simulink model "merge_variable_grain"  (R2023b)
settings: Solver=FixedStepAuto  StartTime=0.0  StopTime=inf  RelTol=1e-3
InitFcn:
  | myapp = app3;
StartFcn:
  | blk = 'merge_variable_grain/Biquad Filtering/speed_disp';
  | event = 'PostOutputs';
  | listener = @(app,event) updateGUI(myapp);
  | h = add_exec_event_listener(blk, event, listener);
StopFcn:
  | delete(myapp)
values from neighbouring files (symbols this model uses):
  audio_1 = audio_2_nr    [inizio.m]    (also in load_preset_audio.m; resample_workspace.m = resample(audio_1, f_resample, fs))
  audio_2 = audio_2_nr    [inizio.m]    (also in load_preset_audio.m; resample_workspace.m = resample(audio_2, f_resample, fs2))
  audio_3 = audio_3_nr    [inizio.m]    (also in load_preset_audio.m; resample_workspace.m = resample(audio_3, f_resample, fs3))
  fs = f_resample    [inizio.m]    (also in load_preset_audio.m; resample_workspace.m)
undefined symbols (not defined in the file or in its folder): canChannel, DiscIntNeverNeededParam
libraries: canmsglib x14, canlib x9, dspfdesign x9, dspsnks4 x1, audiofilters x1, audiodynamicrange x1, simulink x1
settings Model: Creator=The MathWorks, Inc.  LastModifiedBy=giorg
settings SolverCC: AlgebraicLoopSolver=TrustRegion
settings DataIOCC: SaveFormat=Array  ReturnWorkspaceOutputs=off
settings DebuggingCC: UnconnectedInputMsg=warning  UnconnectedOutputMsg=warning  UnconnectedLineMsg=warning  ArithmeticOperatorsInVariantConditions=warning
settings ModelReferenceCC: EnableRefExpFcnMdlSchedulingChecks=on
settings SFSimCC: SimUseLocalCustomCode=off  CustomCodeUndefinedFunction=UseInterfaceOnly
settings RTWCC: RTWUseLocalCustomCode=off

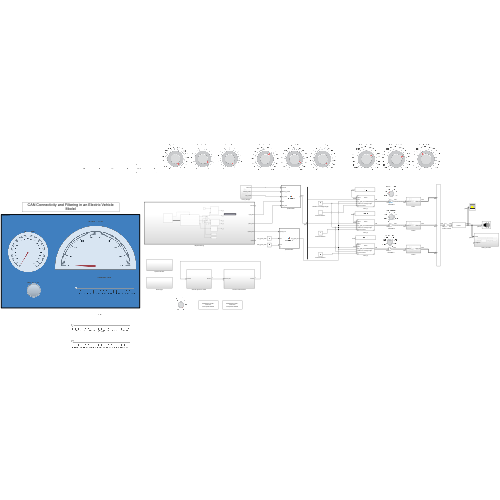
[thumbnail: Simulink's stored preview of the top-level diagram]
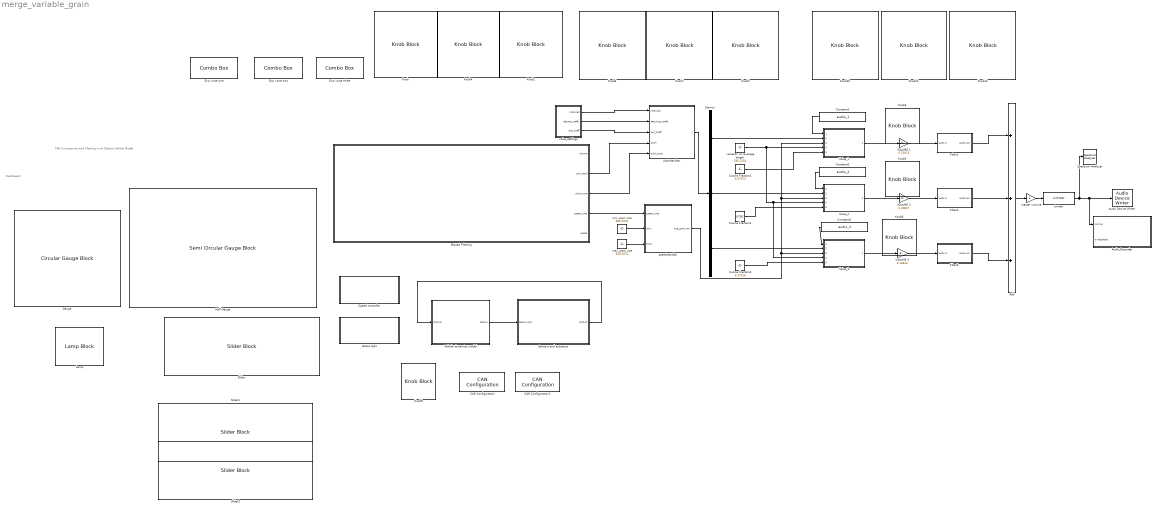
== system merge_variable_grain ==
  note: Dashboard
  note: CAN Connectivity and Filtering in an Electric Vehicle Model
  Add : Sum  Inputs=+++
  Audio Device Writer : dspsnks4/Audio Device Writer  Driver=DirectSound  Device=Default  InheritSampleRate=off  SampleRate=fs  BitDepth=16-bit integer  BufferSize=4096  NumBuffers=10  DefaultOutputChannelMapping=on  OutputChannelMapping=1:2  OutputNumUnderrunSamples=off  DriverIdx=1  DeviceWarnFlag=''
  Audio_Recorder : Subsystem
  Biquad Filtering : Subsystem  TreatAsAtomicUnit=on
  Brake light : Subsystem
  CAN Configuration : canlib/CAN Configuration  BlockHandle=142.0001  Device=MathWorks Virtual 1 (Channel 1)  DeviceMenu=MathWorks Virtual 1 (Channel 1)  ObjConstructor=canChannel('MathWorks', 'Virtual 1', 1)  BusSpeed=500000  EnableBitParameters=off  AckMode=Normal
  CAN Configuration1 : canlib/CAN Configuration  BlockHandle=143.0001  Device=MathWorks Virtual 1 (Channel 2)  DeviceMenu=MathWorks Virtual 1 (Channel 2)  ObjConstructor=canChannel('MathWorks', 'Virtual 1', 2)  BusSpeed=500000  EnableBitParameters=off  AckMode=Normal
  Constant1 : Constant  Value=audio_1
  Constant2 : Constant  Value=audio_2
  Constant3 : Constant  Value=audio_3
  Cosine Fraction1 : Constant  Value=0.67973
  Cosine Fraction2 : Constant  Value=0.7202
  Cosine Fraction3 : Constant  Value=0.37916
  Demux : Demux  Outputs=3
  Exp voice one : ComboBox  LabelPosition=Hide  SelectedLabel=Linear
      settings: Values={{'Linear', 'Quadratic', 'Cubic'}, [1 2 3]}
  Exp voice three : ComboBox  LabelPosition=Hide  SelectedLabel=Linear
      settings: Values={{'Linear', 'Quadratic', 'Cubic'}, [1 2 3]}
  Exp voice two : ComboBox  LabelPosition=Hide  SelectedLabel=Linear
      settings: Values={{'Linear', 'Quadratic', 'Cubic'}, [1 2 3]}
  Filter1 : Subsystem
  Filter2 : Subsystem
  Filter3 : Subsystem
  Gauge : CircularGaugeBlock  ScaleMax=200  TickInterval=10
  Half Gauge : SemiCircularGaugeBlock  ScaleMax=9000  TickInterval=1000
  Knob{,3,5,8,10..12} (7 alike) : KnobBlock  ScaleMax=1
  Knob1 : KnobBlock  ScaleMax=12  TickInterval=1
  Knob2 : KnobBlock  ScaleMin=30  ScaleMax=200
  Knob4 : KnobBlock  ScaleMin=-12  ScaleMax=2  TickInterval=1
  Knob6 : KnobBlock  ScaleMin=100  ScaleMax=1000
  Knob7 : KnobBlock  ScaleMin=300  ScaleMax=1000
  Knob9 : KnobBlock  ScaleMin=0.5  ScaleMax=1
  Lamp : LampBlock
  Limiter : audiodynamicrange/Limiter  ThresholdPort=off  Threshold=0  KneeWidthPort=off  KneeWidth=0.0  AttackTimePort=off  AttackTime=0.0  ReleaseTimePort=off  ReleaseTime=0.120  MakeUpGainMode=Property  MakeUpGain=0.0  InheritSampleRate=off  SampleRate=fs  outputGain=off  EnableSidechain=off  SimulateUsing=Code generation
  Sensors and actuators : Subsystem
  Slider : SliderBlock  ScaleMax=200
  Slider1 : SliderBlock  ScaleMax=1
  Slider2 : SliderBlock  ScaleMax=1
  Spectrum Analyzer : SpectrumAnalyzer  WindowPosition=[309.000000,143.000000,800.000000,500.000000,]  Visible=on  ScopeFrameLocation=window  SampleRateSource=Property  SampleRate=44.1e3  PlotAsTwoSidedSpectrum=off  FrequencyScale=Log  FrequencySpan=Start and stop frequencies  StartFrequency=20  StopFrequency=20e3  SpectrumUnits=dBW  YLimits=[-213.94607708,3.88433958]  SelectedToolstripTab=spectrumAnalyzerToolstrip.spectrumTab
  Speed controller : Subsystem
  VOLUME 1 : Gain  Gain=0.31015
  VOLUME 2 : Gain  Gain=0.30827
  VOLUME 3 : Gain  Gain=0.13644
  Vehicle dynamics model : Subsystem
  Voice_1 : Subsystem  ReferencedSubsystem=Voice  rng_seeds=rng_seeds_thread_1  sample_dim_f=max_s1
  Voice_2 : Subsystem  ReferencedSubsystem=Voice  rng_seeds=rng_seeds_thread_2  sample_dim_f=max_s2
  Voice_3 : Subsystem  ReferencedSubsystem=Voice  rng_seeds=rng_seeds_thread_3  sample_dim_f=max_s3
  master volume : Gain
  max_grain_size : Constant  Value=928.4031
  min_grain_size : Constant  Value=665.0231
  pitchHandler : MATLAB Function  TreatAsAtomicUnit=on
  speedHandler : MATLAB Function  TreatAsAtomicUnit=on  mask{fs=fs}
      mask prompts: fs "sampling frequency"
  variation on average length : Constant  Value=195.2254
  voice_settings : Subsystem
  wires:
  Vehicle dynamics model/1(Sensor) -> Sensors and actuators/1(Sensor port)
  Sensors and actuators/1(Control) -> Vehicle dynamics model/1(Control)
  pitchHandler/1(y) -> Demux/1
  Add/1 -> master volume/1
  Voice_1/1 -> VOLUME 1/1
  Demux/1 -> Voice_1/2
  Voice_3/1 -> VOLUME 3/1
  Constant1/1 -> Voice_1/1
  speedHandler/1(avg_grain_len) -> Voice_2/3, Voice_1/3, Voice_3/3
  Biquad Filtering/2(rpm_pitch) -> pitchHandler/4(pitch)
  VOLUME 1/1 -> Filter1/1(audio in)
  VOLUME 3/1 -> Filter3/1(audio in)
  VOLUME 2/1 -> Filter2/1(audio in)
  Demux/2 -> Voice_2/2
  Demux/3 -> Voice_3/2
  Biquad Filtering/3(pitch_tune) -> pitchHandler/5(pitch_tune)
  voice_settings/1(intervals) -> pitchHandler/1(intervals)
  voice_settings/2(detune_coeffs) -> pitchHandler/2(detuning_coeffs)
  Filter1/1(audio out) -> Add/1
  Filter2/1(audio out) -> Add/2
  Filter3/1(audio out) -> Add/3
  min_grain_size/1 -> speedHandler/2(tmin)
  Biquad Filtering/4(speed_tune) -> speedHandler/1(speed_tune)
  max_grain_size/1 -> speedHandler/3(tmax)
  variation on average length/1 -> Voice_3/4, Voice_2/4, Voice_1/4
  Constant3/1 -> Voice_3/1
  voice_settings/3(exp_coeff) -> pitchHandler/3(exp_coeff)
  Voice_2/1 -> VOLUME 2/1
  Constant2/1 -> Voice_2/1
  Cosine Fraction1/1 -> Voice_1/5
  Cosine Fraction2/1 -> Voice_2/5
  Cosine Fraction3/1 -> Voice_3/5
  master volume/1 -> Limiter/1
  Limiter/1 -> Spectrum Analyzer/1, Audio_Recorder/1(normal), Audio Device Writer/1

== system merge_variable_grain/Audio_Recorder ==
  normal : Inport
  a-weighted : Inport  Port=2
  Reshape : Reshape
  Reshape1 : Reshape
  To Workspace : ToWorkspace  VariableName=audio_output  SaveFormat=Structure  SampleTime=-1
      settings: Save2DSignal=2-D array (concatenate along first dimension)
  To Workspace1 : ToWorkspace  VariableName=audio_output_A  SaveFormat=Structure  SampleTime=-1
      settings: Save2DSignal=2-D array (concatenate along first dimension)
  Weighting Filter : audiofilters/Weighting Filter  Method=A-weighting  InheritSampleRate=off  SampleRate=fs  SimulateUsing=Code generation  WorkspaceVariableName=myFilt  OverwriteExportVariable=on  MaskClassType=No mask
  wires:
  Weighting Filter/1 -> Reshape/1
  normal/1 -> Reshape1/1
  Reshape1/1 -> To Workspace/1
  a-weighted/1 -> Weighting Filter/1
  Reshape/1 -> To Workspace1/1

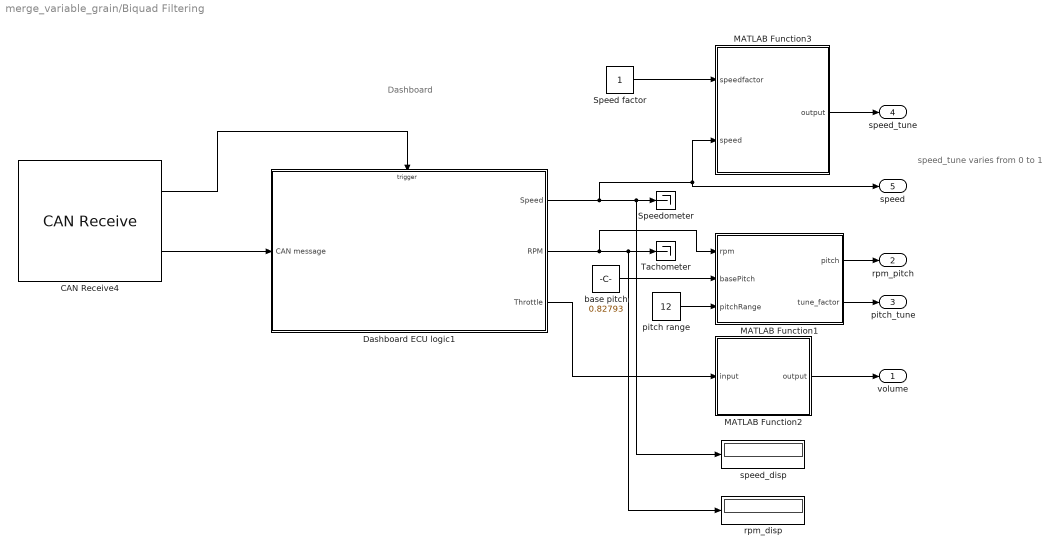
== system merge_variable_grain/Biquad Filtering ==
  note: speed_tune varies from 0 to 1
  note: Dashboard
  CAN Receive4 : canlib/CAN Receive  BlockHandle=19.0001  Device=MathWorks Virtual 1 (Channel 1)  DeviceMenu=MathWorks Virtual 1 (Channel 1)  ObjConstructor=canChannel('MathWorks', 'Virtual 1', 1)  EnableStandardIDsFilter=off  StdIDsCombo=Block all  StandardIDs=0  EnableExtendedIDsFilter=off  ExtIDsCombo=Allow all  ExtendedIDs=[50 100]  SampleTime=0.01  MsgsPerTimestep=all  InternalFilterUpdateStatus=on  BusOutput=on
  Dashboard ECU logic1 : Subsystem  TreatAsAtomicUnit=on
  MATLAB Function1 : MATLAB Function  TreatAsAtomicUnit=on
  MATLAB Function2 : MATLAB Function  TreatAsAtomicUnit=on
  MATLAB Function3 : MATLAB Function  TreatAsAtomicUnit=on
  Speed factor : Constant
  Speedometer : Terminator
  Tachometer : Terminator
  base pitch : Constant  Value=0.82793
  pitch range : Constant  Value=12
  rpm_disp : Display
  speed_disp : Display
  volume : Outport
  rpm_pitch : Outport  Port=2
  pitch_tune : Outport  Port=3
  speed_tune : Outport  Port=4
  speed : Outport  Port=5
  wires:
  Dashboard ECU logic1/3(Throttle) -> MATLAB Function2/1(input)
  MATLAB Function2/1(output) -> volume/1
  Dashboard ECU logic1/1(Speed) -> MATLAB Function3/2(speed), speed/1, speed_disp/1, Speedometer/1
  CAN Receive4/2 -> Dashboard ECU logic1/1(CAN message)
  Dashboard ECU logic1/2(RPM) -> rpm_disp/1, Tachometer/1, MATLAB Function1/1(rpm)
  CAN Receive4/1 -> Dashboard ECU logic1/Trigger
  MATLAB Function1/1(pitch) -> rpm_pitch/1
  MATLAB Function3/1(output) -> speed_tune/1
  Speed factor/1 -> MATLAB Function3/1(speedfactor)
  base pitch/1 -> MATLAB Function1/2(basePitch)
  MATLAB Function1/2(tune_factor) -> pitch_tune/1
  pitch range/1 -> MATLAB Function1/3(pitchRange)

== system merge_variable_grain/Brake light ==
  note: Brake light
  Brake light : Terminator
  Brake light ECU logic : Subsystem  TreatAsAtomicUnit=on
  CAN Receive : canlib/CAN Receive  BlockHandle=137.0001  Device=MathWorks Virtual 1 (Channel 2)  DeviceMenu=MathWorks Virtual 1 (Channel 2)  ObjConstructor=canChannel('MathWorks', 'Virtual 1', 2)  EnableStandardIDsFilter=off  StdIDsCombo=Allow all  StandardIDs=0  EnableExtendedIDsFilter=off  ExtIDsCombo=Allow all  ExtendedIDs=0  SampleTime=0.01  MsgsPerTimestep=all  InternalFilterUpdateStatus=on  BusOutput=on
  wires:
  CAN Receive/1 -> Brake light ECU logic/Trigger
  CAN Receive/2 -> Brake light ECU logic/1(CAN message)
  Brake light ECU logic/1(Brake status) -> Brake light/1

== system merge_variable_grain/Filter1 ==
  audio in : Inport
  Subsystem : Subsystem
  bandwidth : Constant  Value=999
  center_freq : Constant  Value=500
  cutoff_freq : Constant  Value=10000
  switch : Constant
  audio out : Outport
  wires:
  center_freq/1 -> Subsystem/1(In1)
  bandwidth/1 -> Subsystem/2(In2)
  audio in/1 -> Subsystem/3(In3)
  cutoff_freq/1 -> Subsystem/4(In4)
  switch/1 -> Subsystem/5(c)
  Subsystem/1(y) -> audio out/1

== system merge_variable_grain/Filter2 ==
  audio in : Inport
  Subsystem : Subsystem
  bandwidth : Constant  Value=950
  center_freq : Constant  Value=1000
  cutoff_freq : Constant  Value=10000
  switch : Constant
  audio out : Outport
  wires:
  Subsystem/1(y) -> audio out/1
  switch/1 -> Subsystem/5(c)
  cutoff_freq/1 -> Subsystem/4(In4)
  audio in/1 -> Subsystem/3(In3)
  bandwidth/1 -> Subsystem/2(In2)
  center_freq/1 -> Subsystem/1(In1)

== system merge_variable_grain/Filter3 ==
  audio in : Inport
  Subsystem : Subsystem
  bandwidth : Constant  Value=500
  center_freq : Constant  Value=500
  cutoff_freq : Constant  Value=10000
  switch : Constant
  audio out : Outport
  wires:
  center_freq/1 -> Subsystem/1(In1)
  bandwidth/1 -> Subsystem/2(In2)
  audio in/1 -> Subsystem/3(In3)
  cutoff_freq/1 -> Subsystem/4(In4)
  switch/1 -> Subsystem/5(c)
  Subsystem/1(y) -> audio out/1

== system merge_variable_grain/Sensors and actuators ==
  note: Sensors and actuators
  Sensor port : Inport
  Actuators : Subsystem
  CAN Receive interface : Subsystem
  CAN Transmit interface : Subsystem
  Sensors : Subsystem
  Control : Outport  VectorParamsAs1DForOutWhenUnconnected=off
  wires:
  Sensor port/1 -> Sensors/1(Sensor port)
  Sensors/1(RPM) -> CAN Transmit interface/2(RPM)
  Sensors/2(Speed) -> CAN Transmit interface/3(Speed)
  Actuators/1(Control) -> Control/1
  Actuators/2(Brake status) -> CAN Transmit interface/1(Brake status)
  CAN Receive interface/1(Throttle command) -> Actuators/1(Throttle command)
  CAN Receive interface/2(Brake command) -> Actuators/2(Brake command)

== system merge_variable_grain/Speed controller ==
  note: Speed controller
  CAN Receive : canlib/CAN Receive  BlockHandle=455.0001  Device=MathWorks Virtual 1 (Channel 2)  DeviceMenu=MathWorks Virtual 1 (Channel 2)  ObjConstructor=canChannel('MathWorks', 'Virtual 1', 2)  EnableStandardIDsFilter=off  StdIDsCombo=Allow all  StandardIDs=0  EnableExtendedIDsFilter=off  ExtIDsCombo=Allow all  ExtendedIDs=0  SampleTime=0.01  MsgsPerTimestep=all  InternalFilterUpdateStatus=on  BusOutput=on
  Speed controller ECU logic : Subsystem  TreatAsAtomicUnit=on
  wires:
  CAN Receive/1 -> Speed controller ECU logic/Trigger
  CAN Receive/2 -> Speed controller ECU logic/1(CAN message)

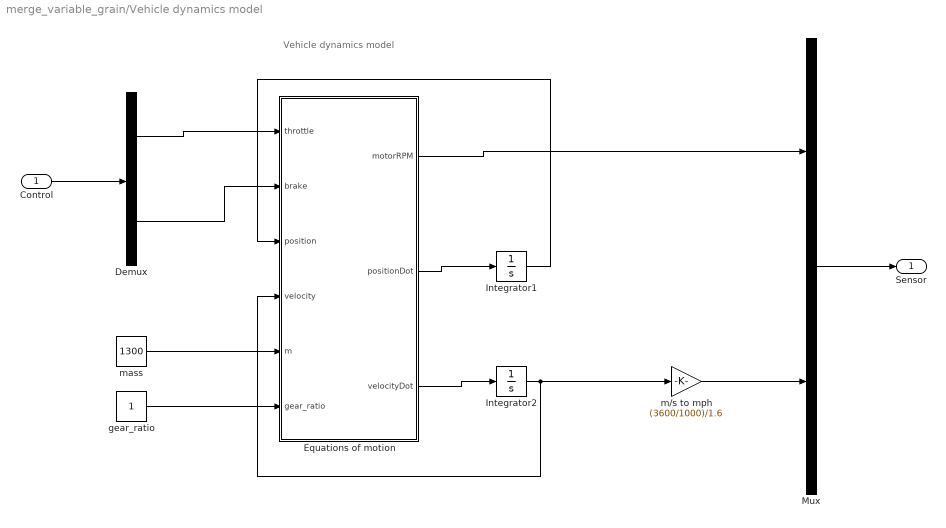
== system merge_variable_grain/Vehicle dynamics model ==
  note: Vehicle dynamics model
  Control : Inport
  Demux : Demux  Outputs=2
  Equations of motion : MATLAB Function  TreatAsAtomicUnit=on
  Integrator1 : Integrator
  Integrator2 : Integrator
  Mux : Mux  Inputs=2
  gear_ratio : Constant
  m/s to mph : Gain  Gain=(3600/1000)/1.6
  mass : Constant  Value=1300
  Sensor : Outport  VectorParamsAs1DForOutWhenUnconnected=off
  wires:
  Demux/1 -> Equations of motion/1(throttle)
  Equations of motion/2(positionDot) -> Integrator1/1
  Equations of motion/3(velocityDot) -> Integrator2/1
  Integrator2/1 -> m/s to mph/1, Equations of motion/4(velocity)
  Integrator1/1 -> Equations of motion/3(position)
  Demux/2 -> Equations of motion/2(brake)
  m/s to mph/1 -> Mux/2
  Equations of motion/1(motorRPM) -> Mux/1
  Control/1 -> Demux/1
  Mux/1 -> Sensor/1
  mass/1 -> Equations of motion/5(m)
  gear_ratio/1 -> Equations of motion/6(gear_ratio)

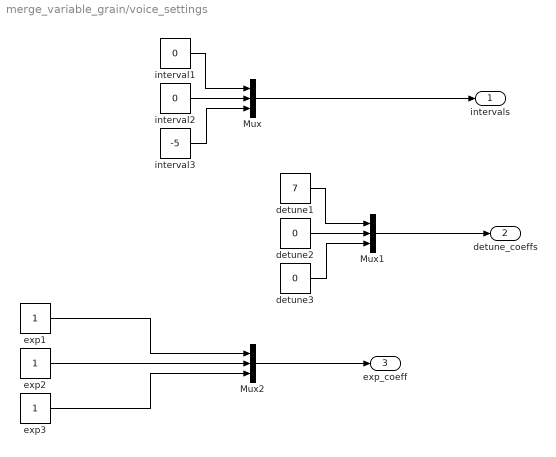
== system merge_variable_grain/voice_settings ==
  Mux : Mux  Inputs=3
  Mux1 : Mux  Inputs=3
  Mux2 : Mux  Inputs=3
  detune1 : Constant  Value=7
  detune2 : Constant  Value=0
  detune3 : Constant  Value=0
  exp1 : Constant
  exp2 : Constant
  exp3 : Constant
  interval1 : Constant  Value=0
  interval2 : Constant  Value=0
  interval3 : Constant  Value=-5
  intervals : Outport
  detune_coeffs : Outport  Port=2
  exp_coeff : Outport  Port=3
  wires:
  interval2/1 -> Mux/2
  interval1/1 -> Mux/1
  interval3/1 -> Mux/3
  Mux/1 -> intervals/1
  detune2/1 -> Mux1/2
  Mux1/1 -> detune_coeffs/1
  detune1/1 -> Mux1/1
  detune3/1 -> Mux1/3
  Mux2/1 -> exp_coeff/1
  exp3/1 -> Mux2/3
  exp2/1 -> Mux2/2
  exp1/1 -> Mux2/1

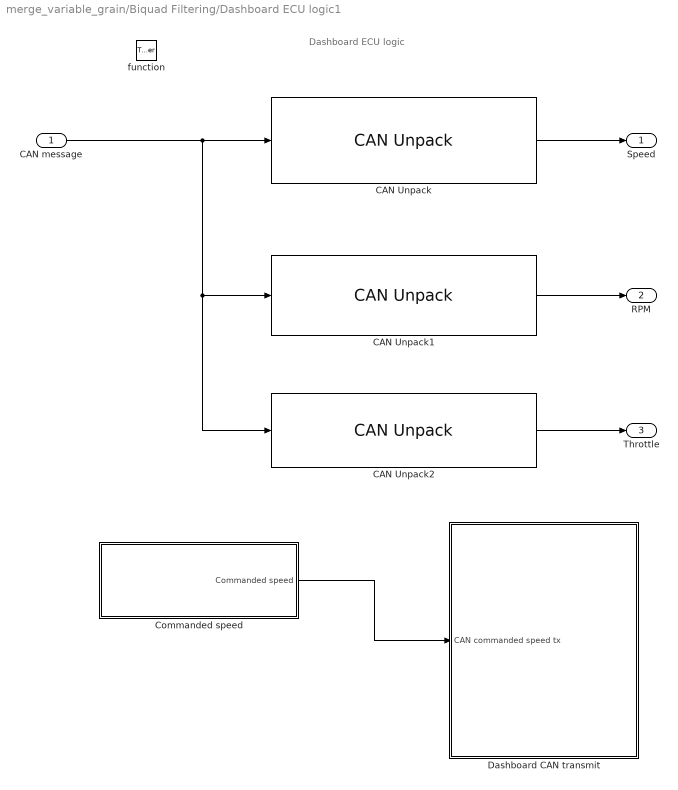
== system merge_variable_grain/Biquad Filtering/Dashboard ECU logic1 ==
  note: Dashboard ECU logic
  CAN message : Inport
  function : TriggerPort  TriggerType=function-call  VariantControl=Variant
  CAN Unpack : canmsglib/CAN Unpack  CANdbFile=canConnectivityForVehicle.dbc  MsgList=SpeedMessage  MsgName=SpeedMessage  MsgIDType=Extended (29-bit identifier)  MsgIdentifier=256  MsgLength=8  SignalInfo={'Speed','0','64','LE','double','Standard','0','1','0','0','100'}  IDPort=off  TimestampPort=off  ErrorPort=off  RemotePort=off  LengthPort=off  StatusPort=off  ApplyMinMax=off
      settings: DataFormat=CANdb specified signals
  CAN Unpack1 : canmsglib/CAN Unpack  CANdbFile=canConnectivityForVehicle.dbc  MsgList=RPMMessage  MsgName=RPMMessage  MsgIDType=Extended (29-bit identifier)  MsgIdentifier=2048  MsgLength=8  SignalInfo={'RPM','0','64','LE','double','Standard','0','1','0','0','10000'}  IDPort=off  TimestampPort=off  ErrorPort=off  RemotePort=off  LengthPort=off  StatusPort=off  ApplyMinMax=off
      settings: DataFormat=CANdb specified signals
  CAN Unpack2 : canmsglib/CAN Unpack  CANdbFile=canConnectivityForVehicle.dbc  MsgList=ThrottleCommandMessage  MsgName=ThrottleCommandMessage  MsgIDType=Extended (29-bit identifier)  MsgIdentifier=96  MsgLength=8  SignalInfo={'ThrottleCommand','0','64','LE','double','Standard','0','1','0','0','1'}  IDPort=off  TimestampPort=off  ErrorPort=off  RemotePort=off  LengthPort=off  StatusPort=off  ApplyMinMax=off
      settings: LibrarySourceBlock=canlib/CAN Unpack  DataFormat=CANdb specified signals
  Commanded speed : Subsystem
  Dashboard CAN transmit : Subsystem
  Speed : Outport  VectorParamsAs1DForOutWhenUnconnected=off
  RPM : Outport  Port=2  VectorParamsAs1DForOutWhenUnconnected=off
  Throttle : Outport  Port=3
  wires:
  CAN message/1 -> CAN Unpack2/1, CAN Unpack1/1, CAN Unpack/1
  Commanded speed/1(Commanded speed) -> Dashboard CAN transmit/1(CAN commanded speed tx)
  CAN Unpack/1 -> Speed/1
  CAN Unpack1/1 -> RPM/1
  CAN Unpack2/1 -> Throttle/1

== system merge_variable_grain/Brake light/Brake light ECU logic ==
  note: Brake light ECU logic
  CAN message : Inport
  function : TriggerPort  TriggerType=function-call  VariantControl=Variant
  CAN Unpack : canmsglib/CAN Unpack  CANdbFile=canConnectivityForVehicle.dbc  MsgList=BrakeStatusMessage  MsgName=BrakeStatusMessage  MsgIDType=Extended (29-bit identifier)  MsgIdentifier=1280  MsgLength=1  SignalInfo={'BrakeStatus','0','1','LE','unsigned','Standard','0','1','0','0','1'}  IDPort=off  TimestampPort=off  ErrorPort=off  RemotePort=off  LengthPort=off  StatusPort=off  ApplyMinMax=off
      settings: DataFormat=CANdb specified signals
  Brake status : Outport  VectorParamsAs1DForOutWhenUnconnected=off
  wires:
  CAN message/1 -> CAN Unpack/1
  CAN Unpack/1 -> Brake status/1

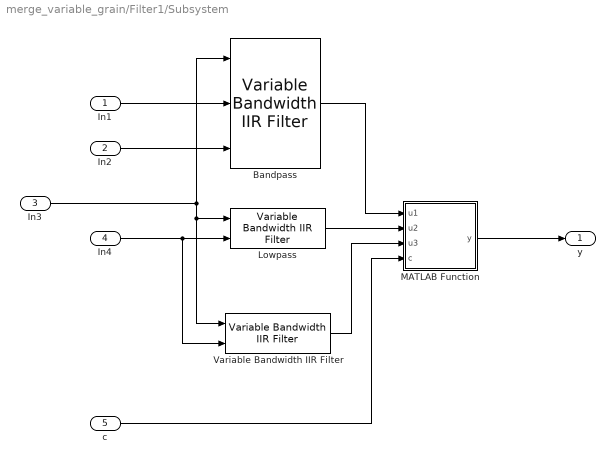
== system merge_variable_grain/Filter1/Subsystem ==
  In1 : Inport
  In2 : Inport  Port=2
  In3 : Inport  Port=3
  In4 : Inport  Port=4
  c : Inport  Port=5
  Bandpass : dspfdesign/Variable Bandwidth IIR Filter  FilterType=Bandpass  FilterOrder=10  PassbandFrequencyPort=on  PassbandFrequency=512  CenterFrequencyPort=on  CenterFrequency=44100/4  BandwidthPort=on  Bandwidth=7680  PassbandRipple=1  StopbandAttenuation=30  SampleRateMode=Specify on dialog  SampleRate=fs  SimulateUsing=Code generation
  Lowpass : dspfdesign/Variable Bandwidth IIR Filter  FilterType=Lowpass  FilterOrder=10  PassbandFrequencyPort=on  PassbandFrequency=512  CenterFrequencyPort=on  CenterFrequency=44100/4  BandwidthPort=on  Bandwidth=7680  PassbandRipple=1  StopbandAttenuation=30  SampleRateMode=Specify on dialog  SampleRate=fs  SimulateUsing=Code generation
  MATLAB Function : MATLAB Function  TreatAsAtomicUnit=on
  Variable Bandwidth IIR Filter : dspfdesign/Variable Bandwidth IIR Filter  FilterType=Highpass  FilterOrder=10  PassbandFrequencyPort=on  PassbandFrequency=512  CenterFrequencyPort=off  CenterFrequency=44100/4  BandwidthPort=off  Bandwidth=7680  PassbandRipple=1  StopbandAttenuation=30  SampleRateMode=Specify on dialog  SampleRate=fs  SimulateUsing=Code generation
  y : Outport
  wires:
  In4/1 -> Variable Bandwidth IIR Filter/2, Lowpass/2
  c/1 -> MATLAB Function/4(c)
  In1/1 -> Bandpass/2
  Lowpass/1 -> MATLAB Function/2(u2)
  In2/1 -> Bandpass/3
  In3/1 -> Variable Bandwidth IIR Filter/1, Lowpass/1, Bandpass/1
  MATLAB Function/1(y) -> y/1
  Bandpass/1 -> MATLAB Function/1(u1)
  Variable Bandwidth IIR Filter/1 -> MATLAB Function/3(u3)

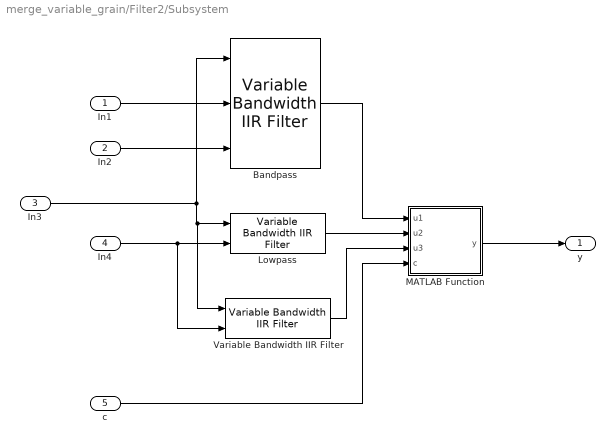
== system merge_variable_grain/Filter2/Subsystem ==
  In1 : Inport
  In2 : Inport  Port=2
  In3 : Inport  Port=3
  In4 : Inport  Port=4
  c : Inport  Port=5
  Bandpass : dspfdesign/Variable Bandwidth IIR Filter  FilterType=Bandpass  FilterOrder=10  PassbandFrequencyPort=on  PassbandFrequency=512  CenterFrequencyPort=on  CenterFrequency=44100/4  BandwidthPort=on  Bandwidth=7680  PassbandRipple=1  StopbandAttenuation=30  SampleRateMode=Specify on dialog  SampleRate=fs2  SimulateUsing=Code generation
  Lowpass : dspfdesign/Variable Bandwidth IIR Filter  FilterType=Lowpass  FilterOrder=10  PassbandFrequencyPort=on  PassbandFrequency=512  CenterFrequencyPort=on  CenterFrequency=44100/4  BandwidthPort=on  Bandwidth=7680  PassbandRipple=1  StopbandAttenuation=30  SampleRateMode=Specify on dialog  SampleRate=fs2  SimulateUsing=Code generation
  MATLAB Function : MATLAB Function  TreatAsAtomicUnit=on
  Variable Bandwidth IIR Filter : dspfdesign/Variable Bandwidth IIR Filter  FilterType=Highpass  FilterOrder=10  PassbandFrequencyPort=on  PassbandFrequency=512  CenterFrequencyPort=off  CenterFrequency=44100/4  BandwidthPort=off  Bandwidth=7680  PassbandRipple=1  StopbandAttenuation=30  SampleRateMode=Specify on dialog  SampleRate=fs  SimulateUsing=Code generation
  y : Outport
  wires:
  Bandpass/1 -> MATLAB Function/1(u1)
  MATLAB Function/1(y) -> y/1
  In3/1 -> Variable Bandwidth IIR Filter/1, Lowpass/1, Bandpass/1
  In2/1 -> Bandpass/3
  Lowpass/1 -> MATLAB Function/2(u2)
  In1/1 -> Bandpass/2
  c/1 -> MATLAB Function/4(c)
  In4/1 -> Variable Bandwidth IIR Filter/2, Lowpass/2
  Variable Bandwidth IIR Filter/1 -> MATLAB Function/3(u3)

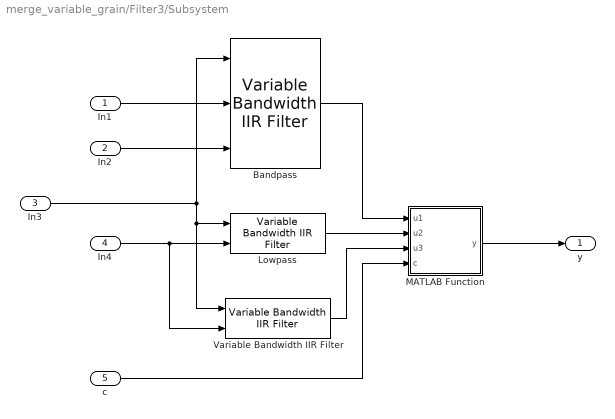
== system merge_variable_grain/Filter3/Subsystem ==
  In1 : Inport
  In2 : Inport  Port=2
  In3 : Inport  Port=3
  In4 : Inport  Port=4
  c : Inport  Port=5
  Bandpass : dspfdesign/Variable Bandwidth IIR Filter  FilterType=Bandpass  FilterOrder=10  PassbandFrequencyPort=on  PassbandFrequency=512  CenterFrequencyPort=on  CenterFrequency=44100/4  BandwidthPort=on  Bandwidth=7680  PassbandRipple=1  StopbandAttenuation=30  SampleRateMode=Specify on dialog  SampleRate=fs3  SimulateUsing=Code generation
  Lowpass : dspfdesign/Variable Bandwidth IIR Filter  FilterType=Lowpass  FilterOrder=10  PassbandFrequencyPort=on  PassbandFrequency=512  CenterFrequencyPort=on  CenterFrequency=44100/4  BandwidthPort=on  Bandwidth=7680  PassbandRipple=1  StopbandAttenuation=30  SampleRateMode=Specify on dialog  SampleRate=fs3  SimulateUsing=Code generation
  MATLAB Function : MATLAB Function  TreatAsAtomicUnit=on
  Variable Bandwidth IIR Filter : dspfdesign/Variable Bandwidth IIR Filter  FilterType=Highpass  FilterOrder=10  PassbandFrequencyPort=on  PassbandFrequency=512  CenterFrequencyPort=off  CenterFrequency=44100/4  BandwidthPort=off  Bandwidth=7680  PassbandRipple=1  StopbandAttenuation=30  SampleRateMode=Specify on dialog  SampleRate=fs  SimulateUsing=Code generation
  y : Outport
  wires:
  In4/1 -> Variable Bandwidth IIR Filter/2, Lowpass/2
  c/1 -> MATLAB Function/4(c)
  In1/1 -> Bandpass/2
  Lowpass/1 -> MATLAB Function/2(u2)
  In2/1 -> Bandpass/3
  In3/1 -> Bandpass/1, Variable Bandwidth IIR Filter/1, Lowpass/1
  MATLAB Function/1(y) -> y/1
  Bandpass/1 -> MATLAB Function/1(u1)
  Variable Bandwidth IIR Filter/1 -> MATLAB Function/3(u3)

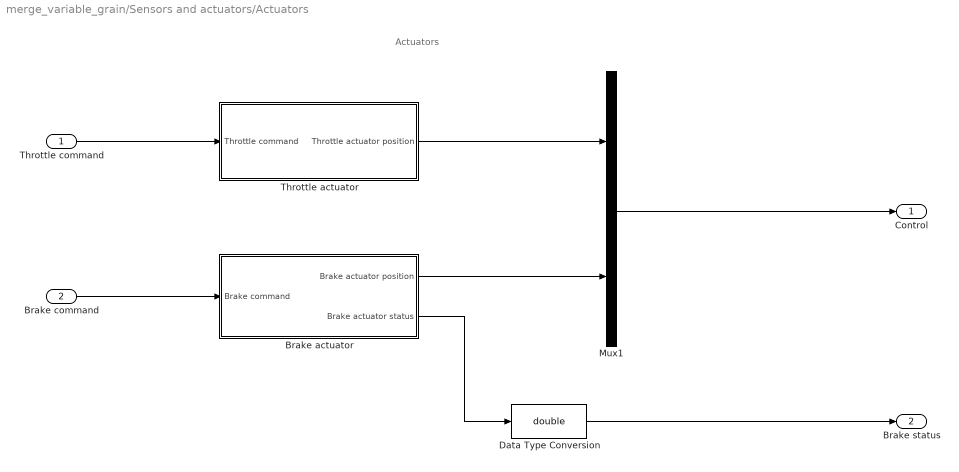
== system merge_variable_grain/Sensors and actuators/Actuators ==
  note: Actuators
  Throttle command : Inport
  Brake command : Inport  Port=2
  Brake actuator : Subsystem
  Data Type Conversion : DataTypeConversion  OutDataTypeStr=double  SaturateOnIntegerOverflow=off  RndMeth=Floor
  Mux1 : Mux  Inputs=2
  Throttle actuator : Subsystem
  Control : Outport  VectorParamsAs1DForOutWhenUnconnected=off
  Brake status : Outport  Port=2  VectorParamsAs1DForOutWhenUnconnected=off
  wires:
  Brake actuator/1(Brake actuator position) -> Mux1/2
  Throttle actuator/1(Throttle actuator position) -> Mux1/1
  Brake command/1 -> Brake actuator/1(Brake command)
  Throttle command/1 -> Throttle actuator/1(Throttle command)
  Data Type Conversion/1 -> Brake status/1
  Brake actuator/2(Brake actuator status) -> Data Type Conversion/1
  Mux1/1 -> Control/1

== system merge_variable_grain/Sensors and actuators/CAN Receive interface ==
  note: CAN Receive interface
  CAN Receive : canlib/CAN Receive  BlockHandle=378.0001  Device=MathWorks Virtual 1 (Channel 1)  DeviceMenu=MathWorks Virtual 1 (Channel 1)  ObjConstructor=canChannel('MathWorks', 'Virtual 1', 1)  EnableStandardIDsFilter=off  StdIDsCombo=Allow all  StandardIDs=0  EnableExtendedIDsFilter=off  ExtIDsCombo=Allow all  ExtendedIDs=0  SampleTime=0.01  MsgsPerTimestep=all  InternalFilterUpdateStatus=off  BusOutput=on
  Extract message : Subsystem  TreatAsAtomicUnit=on
  Throttle command : Outport  VectorParamsAs1DForOutWhenUnconnected=off
  Brake command : Outport  Port=2  VectorParamsAs1DForOutWhenUnconnected=off
  wires:
  CAN Receive/1 -> Extract message/Trigger
  CAN Receive/2 -> Extract message/1(In1)
  Extract message/1(Throttle command) -> Throttle command/1
  Extract message/2(Brake actuator position) -> Brake command/1

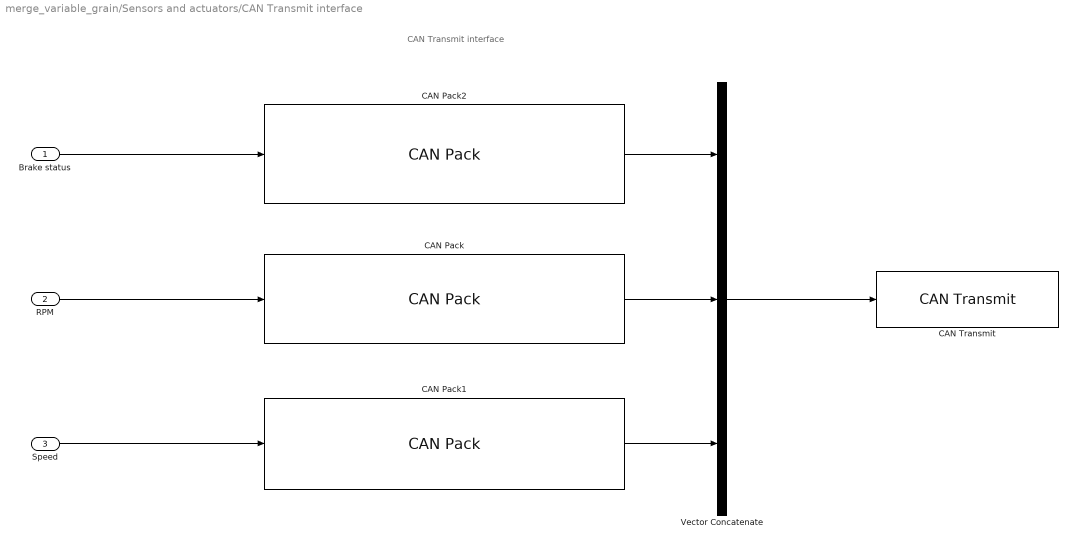
== system merge_variable_grain/Sensors and actuators/CAN Transmit interface ==
  note: CAN Transmit interface
  Brake status : Inport
  RPM : Inport  Port=2
  Speed : Inport  Port=3
  CAN Pack : canmsglib/CAN Pack  CANdbFile=canConnectivityForVehicle.dbc  MsgList=RPMMessage  MsgName=RPMMessage  MsgIDType=Extended (29-bit identifier)  MsgIdentifier=2048  MsgLength=8  Remote=off  ApplyMinMax=off  BusOutput=on  SignalInfo={'RPM','0','64','LE','double','Standard','0','1','0','0','10000'}
      settings: DataFormat=CANdb specified signals
  CAN Pack1 : canmsglib/CAN Pack  CANdbFile=canConnectivityForVehicle.dbc  MsgList=SpeedMessage  MsgName=SpeedMessage  MsgIDType=Extended (29-bit identifier)  MsgIdentifier=256  MsgLength=8  Remote=off  ApplyMinMax=off  BusOutput=on  SignalInfo={'Speed','0','64','LE','double','Standard','0','1','0','0','100'}
      settings: DataFormat=CANdb specified signals
  CAN Pack2 : canmsglib/CAN Pack  CANdbFile=canConnectivityForVehicle.dbc  MsgList=BrakeStatusMessage  MsgName=BrakeStatusMessage  MsgIDType=Extended (29-bit identifier)  MsgIdentifier=1280  MsgLength=1  Remote=off  ApplyMinMax=off  BusOutput=on  SignalInfo={'BrakeStatus','0','1','LE','unsigned','Standard','0','1','0','0','1'}
      settings: DataFormat=CANdb specified signals
  CAN Transmit : canlib/CAN Transmit  BlockHandle=406.0001  Device=MathWorks Virtual 1 (Channel 1)  DeviceMenu=MathWorks Virtual 1 (Channel 1)  ObjConstructor=canChannel('MathWorks', 'Virtual 1', 1)  EnableEventTransmit=off  EnablePeriodicTransmit=off  MessagePeriod=1.000
  Vector Concatenate : Concatenate  NumInputs=3
  wires:
  Speed/1 -> CAN Pack1/1
  Brake status/1 -> CAN Pack2/1
  CAN Pack1/1 -> Vector Concatenate/3
  Vector Concatenate/1 -> CAN Transmit/1
  CAN Pack/1 -> Vector Concatenate/2
  CAN Pack2/1 -> Vector Concatenate/1
  RPM/1 -> CAN Pack/1

== system merge_variable_grain/Sensors and actuators/Sensors ==
  note: Sensors
  Sensor port : Inport
  Demux : Demux  Outputs=2
  Motor RPM sensor : Subsystem
  Wheel speed sensor : Subsystem
  RPM : Outport  VectorParamsAs1DForOutWhenUnconnected=off
  Speed : Outport  Port=2  VectorParamsAs1DForOutWhenUnconnected=off
  wires:
  Motor RPM sensor/1(Sensed RPM) -> RPM/1
  Wheel speed sensor/1(Sensed Velocity) -> Speed/1
  Demux/1 -> Motor RPM sensor/1(RPM)
  Demux/2 -> Wheel speed sensor/1(Velocity)
  Sensor port/1 -> Demux/1

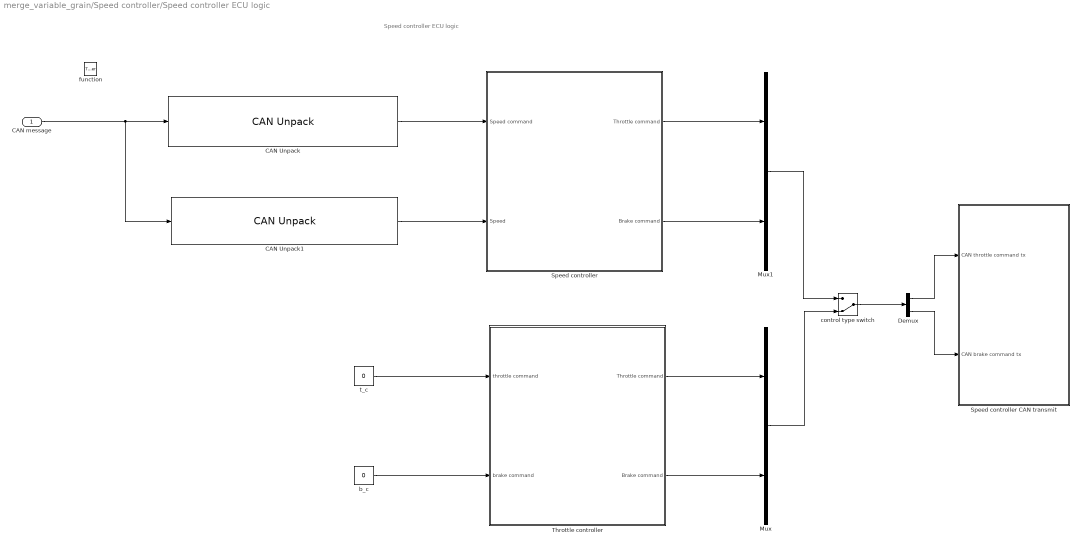
== system merge_variable_grain/Speed controller/Speed controller ECU logic ==
  note: Speed controller ECU logic
  CAN message : Inport
  function : TriggerPort  TriggerType=function-call  VariantControl=Variant
  CAN Unpack : canmsglib/CAN Unpack  CANdbFile=canConnectivityForVehicle.dbc  MsgList=SpeedCommandMessage  MsgName=SpeedCommandMessage  MsgIDType=Extended (29-bit identifier)  MsgIdentifier=1024  MsgLength=8  SignalInfo={'SpeedCommand','0','64','LE','double','Standard','0','1','0','0','100'}  IDPort=off  TimestampPort=off  ErrorPort=off  RemotePort=off  LengthPort=off  StatusPort=off  ApplyMinMax=off
      settings: DataFormat=CANdb specified signals
  CAN Unpack1 : canmsglib/CAN Unpack  CANdbFile=canConnectivityForVehicle.dbc  MsgList=SpeedMessage  MsgName=SpeedMessage  MsgIDType=Extended (29-bit identifier)  MsgIdentifier=256  MsgLength=8  SignalInfo={'Speed','0','64','LE','double','Standard','0','1','0','0','100'}  IDPort=off  TimestampPort=off  ErrorPort=off  RemotePort=off  LengthPort=off  StatusPort=off  ApplyMinMax=off
      settings: DataFormat=CANdb specified signals
  Demux : Demux  Outputs=2
  Mux : Mux  Inputs=2
  Mux1 : Mux  Inputs=2
  Speed controller : Subsystem
  Speed controller CAN transmit : Subsystem
  Throttle controller : Subsystem
  b_c : Constant  Value=0
  control type switch : ManualSwitch  CurrentSetting=0
  t_c : Constant  Value=0
  wires:
  CAN message/1 -> CAN Unpack1/1, CAN Unpack/1
  CAN Unpack/1 -> Speed controller/1(Speed command)
  CAN Unpack1/1 -> Speed controller/2(Speed)
  t_c/1 -> Throttle controller/1(throttle command)
  b_c/1 -> Throttle controller/2(brake command)
  Throttle controller/1(Throttle command) -> Mux/1
  Throttle controller/2(Brake command) -> Mux/2
  Speed controller/1(Throttle command) -> Mux1/1
  Speed controller/2(Brake command) -> Mux1/2
  Mux1/1 -> control type switch/1
  Mux/1 -> control type switch/2
  control type switch/1 -> Demux/1
  Demux/1 -> Speed controller CAN transmit/1(CAN throttle command tx)
  Demux/2 -> Speed controller CAN transmit/2(CAN brake command tx)

== system merge_variable_grain/Biquad Filtering/Dashboard ECU logic1/Commanded speed ==
  note: Commanded speed
  Speed command : Constant  Value=0  OutDataTypeStr=double  SampleTime=Inf
  Zero-Order Hold : ZeroOrderHold  SampleTime=-1
  Commanded speed : Outport  VectorParamsAs1DForOutWhenUnconnected=off
  wires:
  Speed command/1 -> Zero-Order Hold/1
  Zero-Order Hold/1 -> Commanded speed/1

== system merge_variable_grain/Biquad Filtering/Dashboard ECU logic1/Dashboard CAN transmit ==
  note: Dashboard CAN transmit
  CAN commanded speed tx : Inport
  CAN Pack1 : canmsglib/CAN Pack  CANdbFile=canConnectivityForVehicle.dbc  MsgList=SpeedCommandMessage  MsgName=SpeedCommandMessage  MsgIDType=Extended (29-bit identifier)  MsgIdentifier=1024  MsgLength=8  Remote=off  ApplyMinMax=off  BusOutput=on  SignalInfo={'SpeedCommand','0','64','LE','double','Standard','0','1','0','0','100'}
      settings: DataFormat=CANdb specified signals
  CAN Transmit1 : canlib/CAN Transmit  BlockHandle=36.0001  Device=MathWorks Virtual 1 (Channel 1)  DeviceMenu=MathWorks Virtual 1 (Channel 1)  ObjConstructor=canChannel('MathWorks', 'Virtual 1', 1)  EnableEventTransmit=off  EnablePeriodicTransmit=on  MessagePeriod=0.01
  wires:
  CAN commanded speed tx/1 -> CAN Pack1/1
  CAN Pack1/1 -> CAN Transmit1/1

== system merge_variable_grain/Sensors and actuators/Actuators/Brake actuator ==
  note: Brake actuator
  Brake command : Inport
  Brake actuator : TransferFcn  Denominator=[0.1 1]
  Brake status sensor : Subsystem
  Brake actuator position : Outport  VectorParamsAs1DForOutWhenUnconnected=off
  Brake actuator status : Outport  Port=2  VectorParamsAs1DForOutWhenUnconnected=off
  wires:
  Brake status sensor/1(Brake status) -> Brake actuator status/1
  Brake command/1 -> Brake actuator/1
  Brake actuator/1 -> Brake actuator position/1, Brake status sensor/1(Brake actuator position)

== system merge_variable_grain/Sensors and actuators/Actuators/Throttle actuator ==
  note: Throttle actuator
  Throttle command : Inport
  Throttle actuator : TransferFcn  Denominator=[0.1 1]
  Throttle actuator position : Outport  VectorParamsAs1DForOutWhenUnconnected=off
  wires:
  Throttle command/1 -> Throttle actuator/1
  Throttle actuator/1 -> Throttle actuator position/1

== system merge_variable_grain/Sensors and actuators/CAN Receive interface/Extract message ==
  note: Extract message
  In1 : Inport
  function : TriggerPort  TriggerType=function-call  VariantControl=Variant
  CAN Unpack : canmsglib/CAN Unpack  CANdbFile=canConnectivityForVehicle.dbc  MsgList=ThrottleCommandMessage  MsgName=ThrottleCommandMessage  MsgIDType=Extended (29-bit identifier)  MsgIdentifier=96  MsgLength=8  SignalInfo={'ThrottleCommand','0','64','LE','double','Standard','0','1','0','0','1'}  IDPort=off  TimestampPort=off  ErrorPort=off  RemotePort=off  LengthPort=off  StatusPort=off  ApplyMinMax=off
      settings: DataFormat=CANdb specified signals
  CAN Unpack1 : canmsglib/CAN Unpack  CANdbFile=canConnectivityForVehicle.dbc  MsgList=BrakeCommandMessage  MsgName=BrakeCommandMessage  MsgIDType=Extended (29-bit identifier)  MsgIdentifier=81  MsgLength=8  SignalInfo={'BrakeCommand','0','64','LE','double','Standard','0','1','0','0','1'}  IDPort=off  TimestampPort=off  ErrorPort=off  RemotePort=off  LengthPort=off  StatusPort=off  ApplyMinMax=off
      settings: DataFormat=CANdb specified signals
  Throttle command : Outport  VectorParamsAs1DForOutWhenUnconnected=off
  Brake actuator position : Outport  Port=2  VectorParamsAs1DForOutWhenUnconnected=off
  wires:
  In1/1 -> CAN Unpack1/1, CAN Unpack/1
  CAN Unpack/1 -> Throttle command/1
  CAN Unpack1/1 -> Brake actuator position/1

== system merge_variable_grain/Sensors and actuators/Sensors/Motor RPM sensor ==
  note: Motor RPM sensor
  RPM : Inport
  Zero-Order Hold : ZeroOrderHold  SampleTime=.01
  Sensed RPM : Outport  VectorParamsAs1DForOutWhenUnconnected=off
  wires:
  Zero-Order Hold/1 -> Sensed RPM/1
  RPM/1 -> Zero-Order Hold/1

== system merge_variable_grain/Sensors and actuators/Sensors/Wheel speed sensor ==
  note: Wheel speed sensor
  Velocity : Inport
  Zero-Order Hold : ZeroOrderHold  SampleTime=.01
  Sensed Velocity : Outport  VectorParamsAs1DForOutWhenUnconnected=off
  wires:
  Zero-Order Hold/1 -> Sensed Velocity/1
  Velocity/1 -> Zero-Order Hold/1

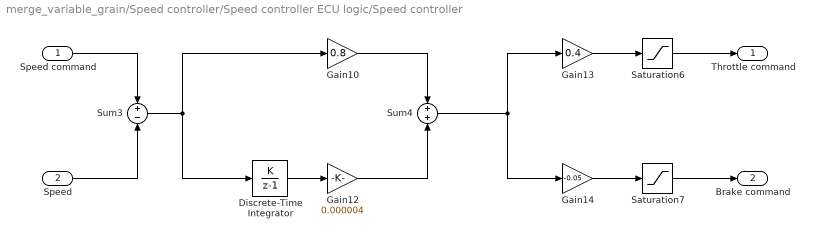
== system merge_variable_grain/Speed controller/Speed controller ECU logic/Speed controller ==
  Speed command : Inport
  Speed : Inport  Port=2
  Discrete-Time Integrator : DiscreteIntegrator  IntegratorMethod=Accumulation: Forward Euler  gainval=1  SampleTime=-1  ICPrevOutput=DiscIntNeverNeededParam  ICPrevScaledInput=DiscIntNeverNeededParam
  Gain10 : Gain  Gain=0.8
  Gain12 : Gain  Gain=0.000004
  Gain13 : Gain  Gain=0.4
  Gain14 : Gain  Gain=-0.05
  Saturation6 : Saturate  UpperLimit=1  LowerLimit=0
  Saturation7 : Saturate  UpperLimit=1  LowerLimit=0
  Sum3 : Sum  Inputs=+|-
  Sum4 : Sum  Inputs=+|+
  Throttle command : Outport  VectorParamsAs1DForOutWhenUnconnected=off
  Brake command : Outport  Port=2  VectorParamsAs1DForOutWhenUnconnected=off
  wires:
  Saturation7/1 -> Brake command/1
  Saturation6/1 -> Throttle command/1
  Speed command/1 -> Sum3/1
  Speed/1 -> Sum3/2
  Sum3/1 -> Discrete-Time Integrator/1, Gain10/1
  Discrete-Time Integrator/1 -> Gain12/1
  Gain10/1 -> Sum4/1
  Sum4/1 -> Gain14/1, Gain13/1
  Gain14/1 -> Saturation7/1
  Gain13/1 -> Saturation6/1
  Gain12/1 -> Sum4/2

== system merge_variable_grain/Speed controller/Speed controller ECU logic/Speed controller CAN transmit ==
  CAN throttle command tx : Inport
  CAN brake command tx : Inport  Port=2
  CAN Pack : canmsglib/CAN Pack  CANdbFile=canConnectivityForVehicle.dbc  MsgList=ThrottleCommandMessage  MsgName=ThrottleCommandMessage  MsgIDType=Extended (29-bit identifier)  MsgIdentifier=96  MsgLength=8  Remote=off  ApplyMinMax=off  BusOutput=on  SignalInfo={'ThrottleCommand','0','64','LE','double','Standard','0','1','0','0','1'}
      settings: DataFormat=CANdb specified signals
  CAN Pack1 : canmsglib/CAN Pack  CANdbFile=canConnectivityForVehicle.dbc  MsgList=BrakeCommandMessage  MsgName=BrakeCommandMessage  MsgIDType=Extended (29-bit identifier)  MsgIdentifier=81  MsgLength=8  Remote=off  ApplyMinMax=off  BusOutput=on  SignalInfo={'BrakeCommand','0','64','LE','double','Standard','0','1','0','0','1'}
      settings: DataFormat=CANdb specified signals
  CAN Transmit : canlib/CAN Transmit  BlockHandle=498.0001  Device=MathWorks Virtual 1 (Channel 1)  DeviceMenu=MathWorks Virtual 1 (Channel 1)  ObjConstructor=canChannel('MathWorks', 'Virtual 1', 1)  EnableEventTransmit=off  EnablePeriodicTransmit=on  MessagePeriod=0.01
  Vector Concatenate : Concatenate
  wires:
  CAN Pack/1 -> Vector Concatenate/1
  CAN throttle command tx/1 -> CAN Pack/1
  CAN brake command tx/1 -> CAN Pack1/1
  CAN Pack1/1 -> Vector Concatenate/2
  Vector Concatenate/1 -> CAN Transmit/1

== system merge_variable_grain/Speed controller/Speed controller ECU logic/Throttle controller ==
  throttle command : Inport
  brake command : Inport  Port=2
  Saturation6 : Saturate  UpperLimit=1  LowerLimit=0
  Saturation7 : Saturate  UpperLimit=1  LowerLimit=0
  Throttle command : Outport  VectorParamsAs1DForOutWhenUnconnected=off
  Brake command : Outport  Port=2  VectorParamsAs1DForOutWhenUnconnected=off
  wires:
  throttle command/1 -> Saturation6/1
  brake command/1 -> Saturation7/1
  Saturation6/1 -> Throttle command/1
  Saturation7/1 -> Brake command/1

== system merge_variable_grain/Sensors and actuators/Actuators/Brake actuator/Brake status sensor ==
  note: Brake status sensor
  Brake actuator position : Inport
  Compare To Constant : simulink/Logic and Bit Operations/Compare To Constant  relop=>  const=0.01  OutDataTypeStr=boolean
  Zero-Order Hold : ZeroOrderHold  SampleTime=0.01
  Brake status : Outport  VectorParamsAs1DForOutWhenUnconnected=off
  wires:
  Zero-Order Hold/1 -> Brake status/1
  Brake actuator position/1 -> Compare To Constant/1
  Compare To Constant/1 -> Zero-Order Hold/1

== matlab function merge_variable_grain/Filter1/Subsystem/MATLAB Function ==
  data: u1 input; y output size=1024; u2 input; u3 input; c input
function y = fcn(u1, u2, u3, c)
y = 0;
if c == 0
    y = u1;
end
if c == 1
    y = u2;
end
if c == 2
    y = u3;
end

== matlab function merge_variable_grain/Vehicle dynamics model/Equations of motion ==
  data: throttle input; brake input; position input; motorRPM output; positionDot output; velocity input; velocityDot output; m input; gear_ratio input
function [motorRPM, positionDot, velocityDot] = car(throttle, brake, position, velocity, m, gear_ratio) %#ok<INUSL>
% This function defines the equations of motion of the vehicle. The vehicle
% is powered by an electric motor with a gearbox. The gear ratio from the
% motor to the wheels is 6:1.

% Radius of wheel
wheelRadius = (195/2)/1000;

% Define the mass properties 
wheelMass = 10;
chassisMass = m;
wheelMomentOfInertia = 0.5*wheelMass*wheelRadius*wheelRadius; 
mass = (4*wheelMass) + chassisMass + (4 * wheelMomentOfInertia/(wheelRadius^2));

% Compute the motor RPM from the wheel speed assuming that the wheels don't
% slip.
motorRPM = (velocity/wheelRadius)*(60/(2*pi))*gear_ratio;    

% Compute the upper bound of the motor torque for the current RPM.
motorTorqueUpperBound = 300*6*exp(-(0.0001*motorRPM));      % 6 is a magic number for now

% Compute the forces acting on the vehicle.
dragForce = 0.5*1.225*(velocity^2)*2; %hava direnci
totalFrictionForce = 0.4*velocity;
motorForce = throttle*motorTorqueUpperBound*gear_ratio/wheelRadius;
brakeForce = brake*sign(velocity)*1600/wheelRadius;
force = motorForce - dragForce - totalFrictionForce - brakeForce; %total hali

% Equations of motion (dot türev demek)
positionDot = velocity; %aracin hizi 
velocityDot = force/mass; %aracin ivmesi

== matlab function merge_variable_grain/Biquad Filtering/MATLAB Function1 ==
  data: rpm input; pitch output; basePitch input; tune_factor output; pitchRange input
function [pitch, tune_factor] = rpmToPitch(rpm, basePitch, pitchRange)
    % Bu değerler örnek olarak verilmiştir ve projenize göre değiştirilmelidir.
    baseFreq = 280; % Hz cinsinden motorun minimum RPM'deki baz frekansı
    maxRPM = 8000;  % Motorun maksimum RPM değeri
    freqRange = 300; % Motorun rölantiden maksimum RPM'ye kadar frekans aralığı
   

    % RPM'den Frekans'a dönüşüm
    freq = baseFreq + (rpm / maxRPM) * freqRange;
    pitch = basePitch + (rpm / maxRPM) * pitchRange;
    tune_factor = rpm/maxRPM;
    if tune_factor > 1
        tune_factor = 1;
end

== matlab function merge_variable_grain/Biquad Filtering/MATLAB Function2 ==
  data: input input; output output
function output = throttleToVolume(input)
% input değeri 0-100 arası olacak şekilde varsayılmıştır.
% output, 0-1 arası bir hacim değerine dönüştürülür.
min = 0.9;
max = 1;

%output = input / 100;
output = (max - min)*input + min;

end

== matlab function merge_variable_grain/Biquad Filtering/MATLAB Function3 ==
  data: speedfactor input; speed input; output output
function output = speedtotune(speedfactor, speed)
    % we want to obtain a tuning factor out of speed
    maxSpeed = 200;

    output = speedfactor * speed/maxSpeed;
end

== matlab function merge_variable_grain/Filter2/Subsystem/MATLAB Function ==
  data: u1 input; y output size=1024; u2 input; u3 input; c input
function y = fcn(u1, u2, u3, c)
y = 0;
if c == 0
    y = u1;
end
if c == 1
    y = u2;
end
if c == 2
   y = u3;
end

== matlab function merge_variable_grain/pitchHandler ==
  data: intervals input; detuning_coeffs input; exp_coeff input; pitch input; y output; pitch_tune input
function y = pitchHandler(intervals, detuning_coeffs, exp_coeff, pitch, pitch_tune)

y = zeros(3,1);

y(1) = pitch^exp_coeff(1);
y(2) = pitch^exp_coeff(2);
y(3) = pitch^exp_coeff(3);

coeff_vector = ones(size(exp_coeff));  % Vector of coefficient 
% When exp is 2 i need to multiply for the sign of the pitch
coeff_vector(mod(exp_coeff, 2) == 0) = sign(pitch);
y = y .* coeff_vector;

y(1) = y(1) + intervals(1) + detuning_coeffs(1) * pitch_tune;
y(2) = y(2) + intervals(2) + detuning_coeffs(2) * pitch_tune;
y(3) = y(3) + intervals(3) + detuning_coeffs(3) * pitch_tune;

== matlab function merge_variable_grain/speedHandler ==
  data: speed_tune input; avg_grain_len output; tmin input; tmax input; fs parameter
% INPUT: value between 0 and 1 that is a relative index of how fast the car
% can go (speed_tune), minimum time duration of the grain in ms(tmin),
% maximum time duration of the grain in ms (tmax), sampling frequency (fs)

% OUTPUT: grain length based on car relative speed (avg_grain_len)

% Function that controls the average length of the grains based on the
% speed
function avg_grain_len = speedHandler(speed_tune, tmin, tmax, fs)
    
    tmin = tmin / 1000; % ms -> s because they need to be converted to samples
    tmax = tmax / 1000;
    min_grain = ceil(tmin / (1/fs));
    max_grain = ceil(tmax / (1/fs));
    y_range = max_grain - min_grain;
    avg_grain_len = max_grain - (speed_tune) * y_range;
end

== matlab function merge_variable_grain/Filter3/Subsystem/MATLAB Function ==
  data: u1 input; y output size=1024; u2 input; u3 input; c input
function y = fcn(u1, u2, u3, c)
y = 0;
if c == 0
    y = u1;
end
if c == 1
    y = u2;
end
if c == 2
    y = u3;
end
